simulink model "synapse_example_circuit"  (R2022a)
settings: Solver=VariableStepAuto  StartTime=0.0  StopTime=20  RelTol=1e-3
model workspace (MAT data in the model file):
  a = 0.15
  gsyn_base = -1
  loss_prob = 0
libraries: neuromorphic_blocks x8
settings Model: Creator=chris  LastModifiedBy=chris

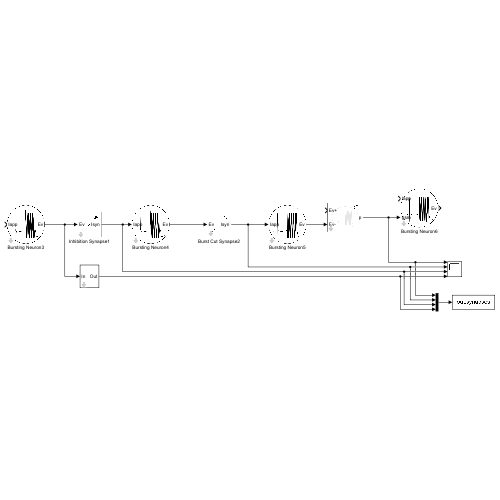
[thumbnail: Simulink's stored preview of the top-level diagram]
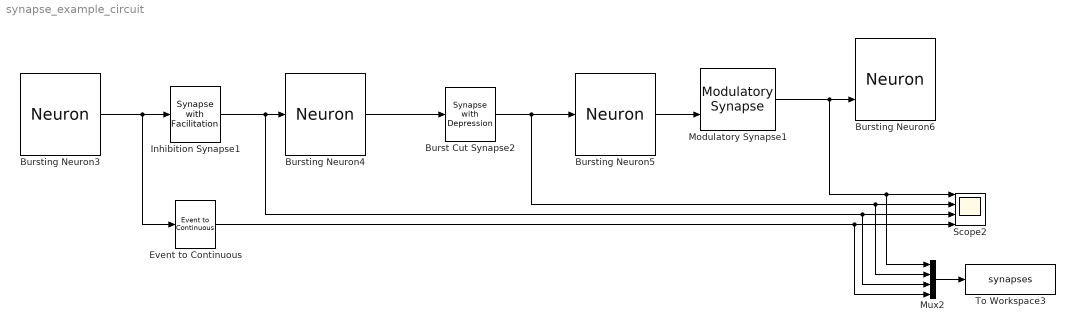
== system synapse_example_circuit ==
  Burst Cut Synapse2 : neuromorphic_blocks/Neural Blocks/Synapse with Depression  gsyn_source=Internal  gsyn=-2  dsyn=5  msyn=10  dsyn_dep=10  msyn_dep=100  timescale=0.004  rel_facilitation=0  rel_depression=100  input=Events  gsyn_in=0  dsyn_in=0  msyn_in=1
      settings: SourceProductName=Neuromorphic Toolbox
  Bursting Neuron3 : neuromorphic_blocks/Neural Blocks/Neuron  gfm_source=Internal  gfm=3  gsp_source=Internal  gsp=6  gsm_source=Internal  gsm=2.5  gup_source=Internal  gup=5  gum_source=Internal  gum=0  dfm=0  dsp=0.5  dsm=-0.5  dup=-0.5  dum=-1  mfm=1  msp=1  msm=1  mup=1  mum=1  timescale=0.004  rel_membrane=0.1  rel_fast=0.1  rel_slow=4  rel_ultraslow=200  Iapp_base=1  V0=-1.2  tresh=0  output=Events
      settings: SourceProductName=Neuromorphic Toolbox
  Bursting Neuron4 : neuromorphic_blocks/Neural Blocks/Neuron  gfm_source=Internal  gfm=3  gsp_source=Internal  gsp=6  gsm_source=Internal  gsm=2.5  gup_source=Internal  gup=5  gum_source=Internal  gum=0  dfm=0  dsp=0.5  dsm=-0.5  dup=-0.5  dum=-1  mfm=1  msp=1  msm=1  mup=1  mum=1  timescale=0.004  rel_membrane=0.1  rel_fast=0.1  rel_slow=4  rel_ultraslow=200  Iapp_base=-1  V0=-1.2  tresh=0  output=Events
      settings: SourceProductName=Neuromorphic Toolbox
  Bursting Neuron5 : neuromorphic_blocks/Neural Blocks/Neuron  gfm_source=Internal  gfm=3  gsp_source=Internal  gsp=6  gsm_source=Internal  gsm=2.5  gup_source=Internal  gup=5  gum_source=Internal  gum=0  dfm=0  dsp=0.5  dsm=-0.5  dup=-0.5  dum=-1  mfm=1  msp=1  msm=1  mup=1  mum=1  timescale=0.004  rel_membrane=0.1  rel_fast=0.1  rel_slow=4  rel_ultraslow=200  Iapp_base=-1  V0=-1.2  tresh=0  output=Events
      settings: SourceProductName=Neuromorphic Toolbox
  Bursting Neuron6 : neuromorphic_blocks/Neural Blocks/Neuron  gfm_source=Internal  gfm=3  gsp_source=Internal  gsp=6  gsm_source=External  gsm=2.5  gup_source=Internal  gup=5  gum_source=Internal  gum=2  dfm=0  dsp=0.5  dsm=-0.5  dup=-0.5  dum=-1  mfm=1  msp=1  msm=1  mup=1  mum=1  timescale=0.004  rel_membrane=0.1  rel_fast=0.1  rel_slow=4  rel_ultraslow=200  Iapp_base=0.05  V0=-1.2  tresh=0  output=Events
      settings: SourceProductName=Neuromorphic Toolbox
  Event to Continuous : neuromorphic_blocks/Events Transmission Blocks/Event to Continuous  gain=1
      settings: SourceProductName=Neuromorphic Toolbox
  Inhibition Synapse1 : neuromorphic_blocks/Neural Blocks/Synapse with Facilitation  gsyn_source=Internal  gsyn=0.2  dsyn=2  msyn=5  timescale=0.004  rel_timescale=10  input=Events  gsyn_in=0  dsyn_in=0  msyn_in=1
      settings: SourceProductName=Neuromorphic Toolbox
  Modulatory Synapse1 : neuromorphic_blocks/Neural Blocks/Modulatory Synapse  base_val=2.5  gsyn_pos_source=Internal  gsyn_pos=1  gsyn_neg_source=Internal  gsyn_neg=1  timescale=0.004  rel_timescale=1000  input=Events  dsyn_pos=0  dsyn_neg=0  msyn_pos=1  msyn_neg=1
      settings: SourceProductName=Neuromorphic Toolbox
  Mux2 : Mux
  Scope2 : Scope  NumInputPorts=4
  To Workspace3 : ToWorkspace  VariableName=synapses  SaveFormat=Structure With Time  SampleTime=-1
  wires:
  Bursting Neuron3/1 -> Event to Continuous/1, Inhibition Synapse1/1
  Bursting Neuron4/1 -> Burst Cut Synapse2/1
  Bursting Neuron5/1 -> Modulatory Synapse1/2
  Mux2/1 -> To Workspace3/1
  Burst Cut Synapse2/1 -> Mux2/2, Scope2/2, Bursting Neuron5/1
  Inhibition Synapse1/1 -> Mux2/3, Scope2/3, Bursting Neuron4/1
  Modulatory Synapse1/1 -> Mux2/1, Scope2/1, Bursting Neuron6/2
  Event to Continuous/1 -> Mux2/4, Scope2/4
